simulink model "Unicycle_1"  (R2017a)
settings: Solver=VariableStepAuto  StartTime=0.0  StopTime=30  RelTol=1e-3
settings Model: Creator=Zichong Lu  LastModifiedBy=Zichong Lu

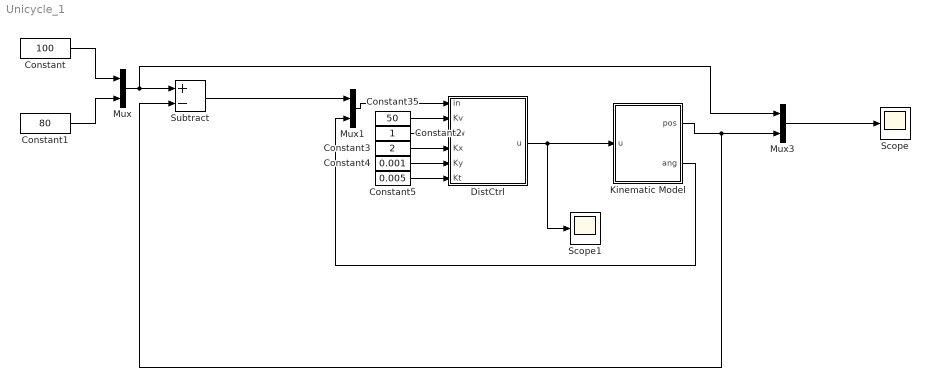
== system Unicycle_1 ==
  Constant : Constant  Value=100
  Constant1 : Constant  Value=80
  Constant2 : Constant
  Constant3 : Constant  Value=2
  Constant35 : Constant  Value=50
  Constant4 : Constant  Value=0.001
  Constant5 : Constant  Value=0.005
  DistCtrl : MATLAB Function  TreatAsAtomicUnit=on
  Kinematic Model : Subsystem
  Mux : Mux  Inputs=2
  Mux1 : Mux  Inputs=2
  Mux3 : Mux  Inputs=2
  Scope : Scope
  Scope1 : Scope
  Subtract : Sum  Inputs=+-
  wires:
  Constant/1 -> Mux/1
  Constant1/1 -> Mux/2
  Mux/1 -> Mux3/1, Subtract/1
  Constant35/1 -> DistCtrl/2(Kv)
  Constant2/1 -> DistCtrl/3(Kw)
  DistCtrl/1(u) -> Scope1/1, Kinematic Model/1(u)
  Mux1/1 -> DistCtrl/1(in)
  Kinematic Model/1(pos) -> Subtract/2, Mux3/2
  Mux3/1 -> Scope/1
  Kinematic Model/2(ang) -> Mux1/2
  Constant5/1 -> DistCtrl/6(Kt)
  Constant3/1 -> DistCtrl/4(Kx)
  Constant4/1 -> DistCtrl/5(Ky)
  Subtract/1 -> Mux1/1

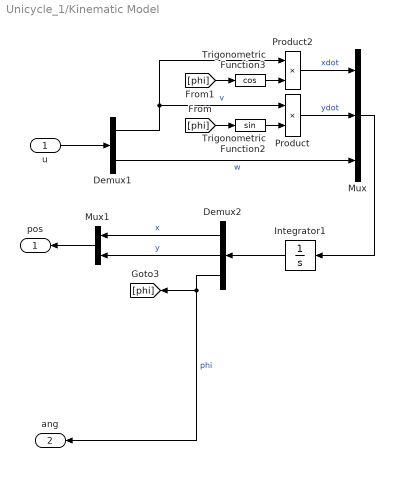
== system Unicycle_1/Kinematic Model ==
  u : Inport
  Demux1 : Demux  Outputs=2
  Demux2 : Demux  Outputs=3
  Integrator1 : Integrator
  Mux : Mux  Inputs=3
  Mux1 : Mux  Inputs=2
  Product : Product
  Product2 : Product
  Trigonometric Function2 : Trigonometry
  Trigonometric Function3 : Trigonometry  Operator=cos
  pos : Outport
  ang : Outport  Port=2
  wires:
  [phi] -> Trigonometric Function3/1
  [phi] -> Trigonometric Function2/1
  Trigonometric Function2/1 -> Product/2
  Trigonometric Function3/1 -> Product2/2
  Mux1/1 -> pos/1
  Demux2/2 -> Mux1/2  "y"
  Demux2/3 -> ang/1, [phi]  "phi"
  u/1 -> Demux1/1
  Product2/1 -> Mux/1  "xdot"
  Demux1/2 -> Mux/3  "w"
  Demux2/1 -> Mux1/1  "x"
  Demux1/1 -> Product2/1, Product/1  "v"
  Integrator1/1 -> Demux2/1
  Product/1 -> Mux/2  "ydot"
  Mux/1 -> Integrator1/1

== matlab function Unicycle_1/DistCtrl ==
  data: in input size=3; u output size=2; Kv input; Kw input; Kx input; Ky input; Kt input
function u   = DistCtrl(in,Kv,Kw,Kx,Ky,Kt)
ex = in(1);
ey = in(2);

% ex = cos(in(3))*in(1)+sin(in(3))*in(2); 
% ey = -sin(in(3))*in(1)+cos(in(3))*in(2); 
theta = in(3);
theta_d = atan2(ey,ex);
et = theta_d - theta; 
vd = sqrt(ex^2+ey^2);
wd = 1/(1+(theta_d)^2);
% Sjavash


% Kb = 0.1;
% v = Kv*vd*cos(et)/(vd+Kb);
% w = -Kw*et;%+wd;

%Luca
% Kx=1.0; 
% Ky=1; 
% Kt=0.01;
u1 = -Kx*ex;
u2 = -Ky*sign(vd)*ey - Kt*et;
v = vd*cos(et)-u1;
w = wd-u2;

%Xi
% K1=1; K2=1; K3=1;
% r=1; d=1; vr=0; wr=0;
% w1 = (vr/r)*cos(et)+(K1/r)*ex+d*wr+r*d*(K2*ey+K3*sin(et));
% w2 = -(vr/r)*cos(et)-(K1/r)*ex+d*wr+r*d*(K2*ey+K3*sin(et));
% v = (w1+w2)/2; w = (w1-w2)/d;
%
u = [v;w];
